simulink model "AC_Vfinal"  (R2019b)
settings: Solver=VariableStepAuto  StartTime=0.0  StopTime=sim_time  RelTol=1e-3
undefined symbols (not defined in the file): a1, A1, a2, A2, Ao, Cp_C, Cp_E, Cpa, Cpe, cpl, cpr, cpr1, cpr2, cpv, D, f1, f2, hfg, hr1, hr2, Kf, Mf, Mfl, Mfv, mr, N, n, Nc, nv, P, Qps, Qs, sp1, Ta, Tin, Uo, V, v, Vh1, Vh2, vs, Wg, Wm
libraries: simulink_extras x13
settings Model: Creator=aravi  LastModifiedBy=aravi
settings DataIOCC: SaveFormat=StructureWithTime  ReturnWorkspaceOutputs=off

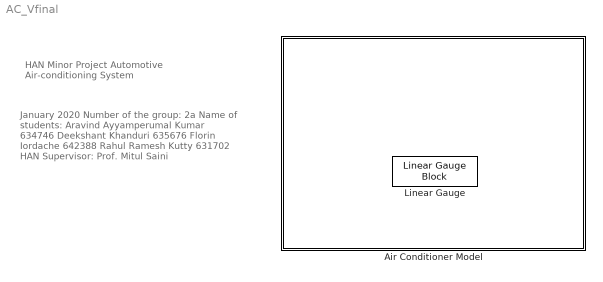
== system AC_Vfinal ==
  note: January 2020
      | Number of the group: 2a
      | Name of students:
      | Aravind Ayyamperumal Kumar 634746
      | Deekshant Khanduri 635676
      | Florin Iordache 642388
      | Rahul Ramesh Kutty 631702
      | HAN Supervisor: Prof. Mitul Saini
  note: HAN Minor Project
      | Automotive Air-conditioning System
  Air Conditioner Model : Subsystem
      mask Display: image('$imagefile'); % Use "Edit Image" on toolstrip to change.
  Linear Gauge : LinearGaugeBlock  ScaleMax=50  TickInterval=5

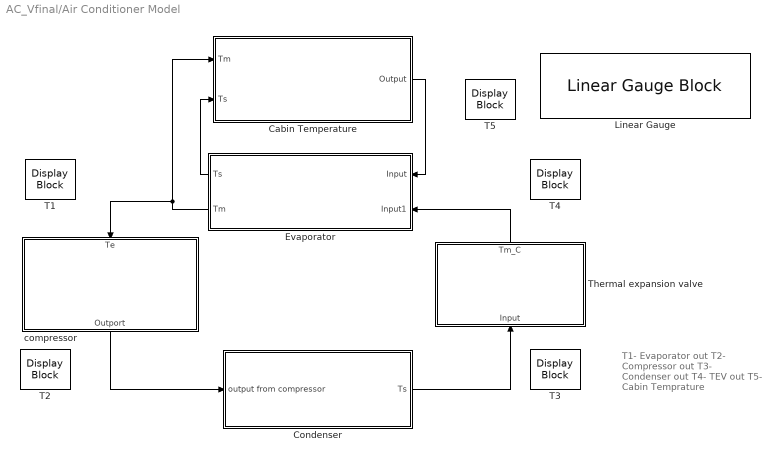
== system AC_Vfinal/Air Conditioner Model ==
  note: T1- Evaporator out
      | T2- Compressor out
      | T3- Condenser out
      | T4- TEV out
      | T5- Cabin Temprature
  Cabin Temperature : Subsystem
      mask Display: image('$imagefile'); % Use "Edit Image" on toolstrip to change.
  Condenser : Subsystem
      mask Display: image('$imagefile'); % Use "Edit Image" on toolstrip to change.
  Evaporator : Subsystem
      mask Display: image('$imagefile'); % Use "Edit Image" on toolstrip to change.
  Linear Gauge : LinearGaugeBlock  ScaleMax=50  TickInterval=5
  T{1..5} (5 alike) : DisplayBlock  LabelPosition=Hide  Format=short  Transparency=1
  Thermal expansion valve : Subsystem
      mask Display: image('$imagefile'); % Use "Edit Image" on toolstrip to change.
  compressor : Subsystem
      mask Display: image('$imagefile'); % Use "Edit Image" on toolstrip to change.
  wires:
  Evaporator/2(Tm) -> compressor/1(Te), Cabin Temperature/1(Tm)
  Condenser/1(Ts) -> Thermal expansion valve/1(Input)
  Cabin Temperature/1(Output) -> Evaporator/1(Input)
  compressor/1(Outport) -> Condenser/1(output from compressor)
  Thermal expansion valve/1(Tm_C) -> Evaporator/2(Input1)
  Evaporator/1(Ts) -> Cabin Temperature/2(Ts)

== system AC_Vfinal/Air Conditioner Model/Cabin Temperature ==
  Tm : Inport
  Ts : Inport  Port=2
  Temperature level : Subsystem
  Output : Outport
  wires:
  Tm/1 -> Temperature level/1(Tm)
  Temperature level/1(Output) -> Output/1
  Ts/1 -> Temperature level/2(Ts)

== system AC_Vfinal/Air Conditioner Model/Condenser ==
  output from compressor : Inport
  Mref : Subsystem
  Td block : Subsystem
  Tm block : Subsystem
  Ts block : Subsystem
  Tw block : Subsystem
  Ts : Outport
  wires:
  Ts block/2(Ts) -> Tw block/1(Ts)
  Tw block/1(Tw) -> Ts block/2(Tw), Td block/1(Tw)
  Td block/1(Td) -> Tw block/4(Td), Ts block/1(Td1)
  Ts block/1(Output to cabin Ts) -> Ts/1
  Tm block/1(Tm_C) -> Tw block/3(Tm), Td block/2(Tm)
  output from compressor/1 -> Tm block/1(Input)
  Mref/1(Out1) -> Tw block/2(Mref)

== system AC_Vfinal/Air Conditioner Model/Evaporator ==
  Input : Inport
  Input1 : Inport  Port=2
  Mref : Subsystem
  Td block : Subsystem
  Tm block : Subsystem
  Ts block : Subsystem
  Tw block : Subsystem
  Ts : Outport
  Tm : Outport  Port=2
  wires:
  Ts block/2(Ts) -> Tw block/1(Ts)
  Td block/1(Td) -> Tw block/4(Td), Ts block/1(Td1)
  Tw block/1(Tw) -> Ts block/2(Tw), Td block/1(Tw)
  Ts block/1(Output to cabin Ts) -> Ts/1
  Tm block/1(Tm_C) -> Tm/1, Tw block/3(Tm), Td block/2(Tm)
  Input/1 -> Tm block/1(Input)
  Input1/1 -> Tm block/2(Input1)
  Mref/1(Out1) -> Tw block/2(Mref)

== system AC_Vfinal/Air Conditioner Model/Thermal expansion valve ==
  note: Differential Equation
  note: Transfer Funtion
  note: Input
  note: process
  note: Output
  note: Input
  note: Process
  note: Output
  note: TinMfvcpv-ToutMflcpl = 0
  Input : Inport
  Gain1 : Gain  Gain=1/(Mfv*cpv)
  Gain4 : Gain  Gain=Mfl*cpl
  Input1 : InportShadow
  Scope : Scope
  Scope2 : Scope
  Transfer Fcn : TransferFcn  Numerator=[Mfl*cpl]  Denominator=[Mfv*cpv]
  Tm_C : Outport
  wires:
  Gain1/1 -> Scope2/1, Tm_C/1
  Input/1 -> Gain4/1
  Gain4/1 -> Gain1/1
  Transfer Fcn/1 -> Scope/1
  Input1/1 -> Transfer Fcn/1

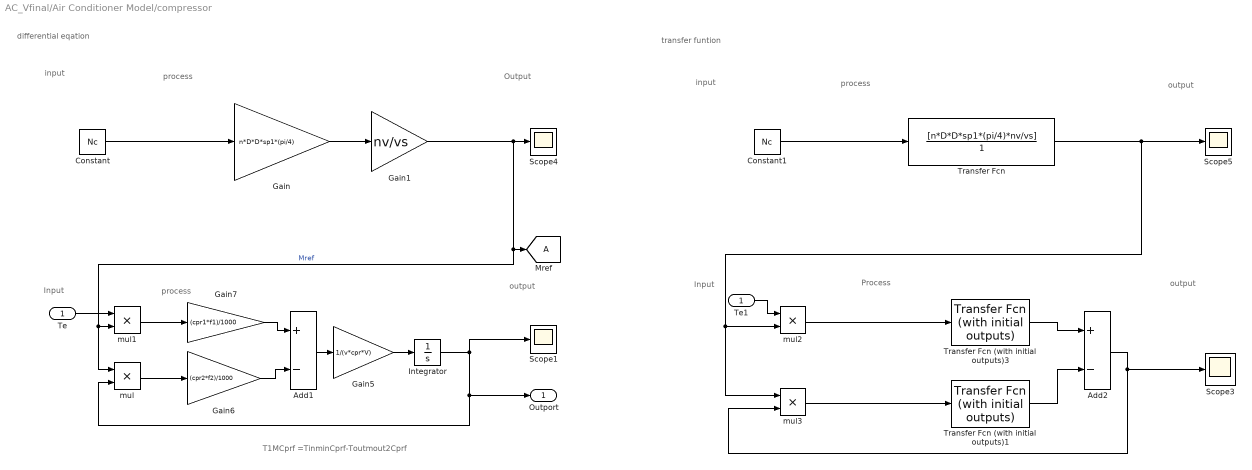
== system AC_Vfinal/Air Conditioner Model/compressor ==
  note: transfer funtion
  note: output
  note: process
  note: input
  note: output
  note: Process
  note: Input
  note: differential eqation
  note: input
  note: process
  note: Output
  note: process
  note: Input
  note: output
  note: T1MCprf =TinminCprf-Toutmout2Cprf
  Te : Inport
  Add1 : Sum  Inputs=+-
  Add2 : Sum  Inputs=+-
  Constant : Constant  Value=Nc  VectorParams1D=off  SampleTime=-1
  Constant1 : Constant  Value=Nc  VectorParams1D=off  SampleTime=-1
  Gain : Gain  Gain=n*D*D*sp1*(pi/4)
  Gain1 : Gain  Gain=nv/vs
  Gain5 : Gain  Gain=1/(v*cpr*V)
  Gain6 : Gain  Gain=(cpr2*f2)/1000
  Gain7 : Gain  Gain=(cpr1*f1)/1000
  Integrator : Integrator  InitialCondition=10
  Scope{1,3..5} (4 alike) : Scope
  Te1 : InportShadow
  Transfer Fcn : TransferFcn  Numerator=[n*D*D*sp1*(pi/4)*nv/vs]  Denominator=[1]
  Transfer Fcn (with initial outputs)1 : simulink_extras/Additional Linear/Transfer Fcn (with initial outputs)  N=[(cpr2*f2)/1000]  D=[v*cpr*V 0]  Y0=10  U0=27
  Transfer Fcn (with initial outputs)3 : simulink_extras/Additional Linear/Transfer Fcn (with initial outputs)  N=[(cpr1*f1)/1000]  D=[v*cpr*V 0]  Y0=20  U0=27
  mul{,1..3} (4 alike) : Product  Inputs=**
  Outport : Outport
  tag scope: A=global
  wires:
  Gain/1 -> Gain1/1
  Constant/1 -> Gain/1
  Integrator/1 -> Scope1/1, mul/2, Outport/1
  Add1/1 -> Gain5/1
  Gain6/1 -> Add1/2
  Gain7/1 -> Add1/1
  mul1/1 -> Gain7/1
  Gain5/1 -> Integrator/1
  Te/1 -> mul1/1
  Gain1/1 -> Scope4/1, [A], mul/1, mul1/2  "Mref"
  mul/1 -> Gain6/1
  Constant1/1 -> Transfer Fcn/1
  Transfer Fcn/1 -> Scope5/1, mul3/1, mul2/2
  mul2/1 -> Transfer Fcn (with initial outputs)3/1
  mul3/1 -> Transfer Fcn (with initial outputs)1/1
  Te1/1 -> mul2/1
  Transfer Fcn (with initial outputs)3/1 -> Add2/1
  Transfer Fcn (with initial outputs)1/1 -> Add2/2
  Add2/1 -> mul3/2, Scope3/1

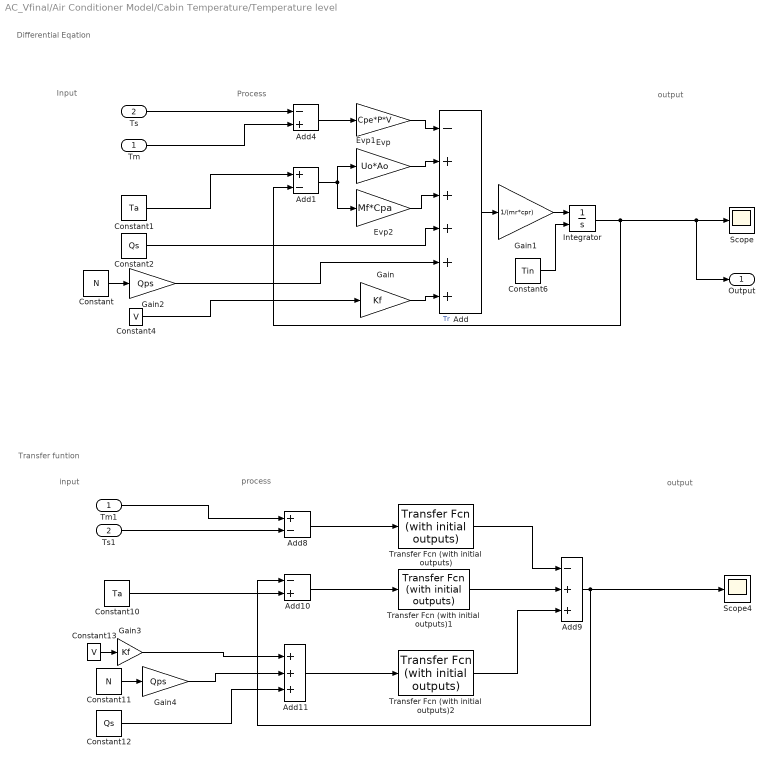
== system AC_Vfinal/Air Conditioner Model/Cabin Temperature/Temperature level ==
  note: Differential Eqation
  note: Input
  note: Process
  note: output
  note: Transfer funtion
  note: input
  note: process
  note: output
  Tm : Inport
  Ts : Inport  Port=2
  Add : Sum  Inputs=-+++++
  Add1 : Sum  Inputs=+-
  Add10 : Sum  Inputs=-+
  Add11 : Sum  Inputs=+++
  Add4 : Sum  Inputs=-+
  Add8 : Sum  Inputs=+-
  Add9 : Sum  Inputs=-++
  Constant : Constant  Value=N
  Constant1 : Constant  Value=Ta
  Constant10 : Constant  Value=Ta
  Constant11 : Constant  Value=N
  Constant12 : Constant  Value=Qs
  Constant13 : Constant  Value=V
  Constant2 : Constant  Value=Qs
  Constant4 : Constant  Value=V
  Constant6 : Constant  Value=Tin
  Evp : Gain  Gain=Cpe*P*V
  Evp1 : Gain  Gain=Uo*Ao
  Evp2 : Gain  Gain=Mf*Cpa
  Gain : Gain  Gain=Kf
  Gain1 : Gain  Gain=1/(mr*cpr)
  Gain2 : Gain  Gain=Qps
  Gain3 : Gain  Gain=Kf
  Gain4 : Gain  Gain=Qps
  Integrator : Integrator  InitialConditionSource=external
  Scope : Scope
  Scope4 : Scope
  Tm1 : InportShadow
  Transfer Fcn (with initial outputs) : simulink_extras/Additional Linear/Transfer Fcn (with initial outputs)  N=[Cpe*V*P]  D=[(mr*cpr) 0 ]  Y0=0  U0=27
  Transfer Fcn (with initial outputs)1 : simulink_extras/Additional Linear/Transfer Fcn (with initial outputs)  N=[Uo*Ao+Mf*Cpa]  D=[(mr*cpr) 0]  Y0=13.5  U0=28
  Transfer Fcn (with initial outputs)2 : simulink_extras/Additional Linear/Transfer Fcn (with initial outputs)  N=[1]  D=[(mr*cpr) 0 ]  Y0=13.5  U0=28
  Ts1 : InportShadow  Port=2
  Output : Outport
  wires:
  Gain1/1 -> Integrator/1
  Constant2/1 -> Add/4
  Constant4/1 -> Gain/1
  Constant/1 -> Gain2/1
  Constant6/1 -> Integrator/2
  Evp1/1 -> Add/2
  Evp2/1 -> Add/3
  Gain/1 -> Add/6
  Evp/1 -> Add/1
  Add/1 -> Gain1/1
  Integrator/1 -> Add1/2, Output/1, Scope/1  "Tr"
  Add1/1 -> Evp2/1, Evp1/1
  Add4/1 -> Evp/1
  Constant1/1 -> Add1/1
  Tm/1 -> Add4/2
  Ts/1 -> Add4/1
  Gain3/1 -> Add11/1
  Transfer Fcn (with initial outputs)1/1 -> Add9/2
  Transfer Fcn (with initial outputs)/1 -> Add9/1
  Constant12/1 -> Add11/3
  Constant13/1 -> Gain3/1
  Transfer Fcn (with initial outputs)2/1 -> Add9/3
  Constant11/1 -> Gain4/1
  Add8/1 -> Transfer Fcn (with initial outputs)/1
  Tm1/1 -> Add8/1
  Ts1/1 -> Add8/2
  Add10/1 -> Transfer Fcn (with initial outputs)1/1
  Add9/1 -> Scope4/1, Add10/1
  Add11/1 -> Transfer Fcn (with initial outputs)2/1
  Constant10/1 -> Add10/2
  Gain2/1 -> Add/5
  Gain4/1 -> Add11/2

== system AC_Vfinal/Air Conditioner Model/Condenser/Mref ==
  Multiply : Gain  Gain=1/10
  Out1 : Outport
  wires:
  [A] -> Multiply/1
  Multiply/1 -> Out1/1

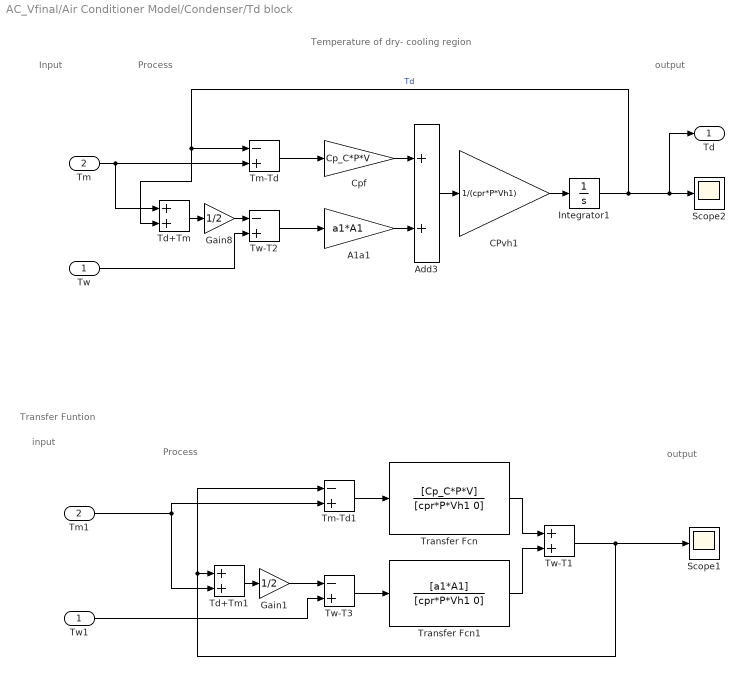
== system AC_Vfinal/Air Conditioner Model/Condenser/Td block ==
  note: Transfer Funtion
  note: output
  note: Process
  note: input
  note: Input
  note: Process
  note: output
  note: Temperature of dry- cooling region
  Tw : Inport
  Tm : Inport  Port=2
  A1a1 : Gain  Gain=a1*A1
  Add3 : Sum
  CPvh1 : Gain  Gain=1/(cpr*P*Vh1)
  Cpf : Gain  Gain=Cp_C*P*V
  Gain1 : Gain  Gain=1/2
  Gain8 : Gain  Gain=1/2
  Integrator1 : Integrator
  Scope1 : Scope
  Scope2 : Scope
  Td+Tm : Sum
  Td+Tm1 : Sum
  Tm-Td : Sum  Inputs=-+
  Tm-Td1 : Sum  Inputs=-+
  Tm1 : InportShadow  Port=2
  Transfer Fcn : TransferFcn  Numerator=[Cp_C*P*V]  Denominator=[cpr*P*Vh1 0]
  Transfer Fcn1 : TransferFcn  Numerator=[a1*A1]  Denominator=[cpr*P*Vh1 0]
  Tw-T1 : Sum
  Tw-T2 : Sum  Inputs=-+
  Tw-T3 : Sum  Inputs=-+
  Tw1 : InportShadow
  Td : Outport
  wires:
  Gain8/1 -> Tw-T2/1
  CPvh1/1 -> Integrator1/1
  Cpf/1 -> Add3/1
  Td+Tm/1 -> Gain8/1
  Tm-Td/1 -> Cpf/1
  Add3/1 -> CPvh1/1
  Integrator1/1 -> Td+Tm/2, Tm-Td/1, Td/1, Scope2/1  "Td"
  A1a1/1 -> Add3/2
  Tw-T2/1 -> A1a1/1
  Tw/1 -> Tw-T2/2
  Tm/1 -> Td+Tm/1, Tm-Td/2
  Transfer Fcn/1 -> Tw-T1/1
  Transfer Fcn1/1 -> Tw-T1/2
  Tw-T1/1 -> Tm-Td1/1, Td+Tm1/1, Scope1/1
  Tw-T3/1 -> Transfer Fcn1/1
  Tm-Td1/1 -> Transfer Fcn/1
  Gain1/1 -> Tw-T3/1
  Td+Tm1/1 -> Gain1/1
  Tw1/1 -> Tw-T3/2
  Tm1/1 -> Tm-Td1/2, Td+Tm1/2

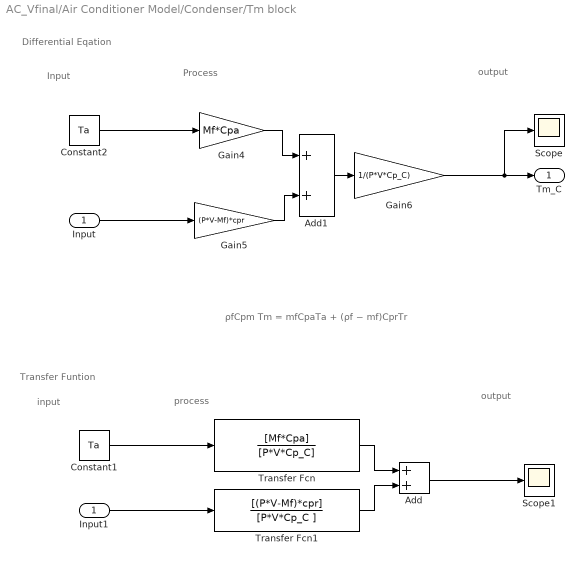
== system AC_Vfinal/Air Conditioner Model/Condenser/Tm block ==
  note: Differential Eqation
  note: Transfer Funtion
  note: output
  note: process
  note: input
  note: Process
  note: ρfCpm Tm = mfCpaTa + (ρf − mf)CprTr
  note: output
  note: Input
  Input : Inport
  Add : Sum
  Add1 : Sum
  Constant1 : Constant  Value=Ta
  Constant2 : Constant  Value=Ta
  Gain4 : Gain  Gain=Mf*Cpa
  Gain5 : Gain  Gain=(P*V-Mf)*cpr
  Gain6 : Gain  Gain=1/(P*V*Cp_C)
  Input1 : InportShadow
  Scope : Scope
  Scope1 : Scope
  Transfer Fcn : TransferFcn  Numerator=[Mf*Cpa]  Denominator=[P*V*Cp_C]
  Transfer Fcn1 : TransferFcn  Numerator=[(P*V-Mf)*cpr]  Denominator=[P*V*Cp_C ]
  Tm_C : Outport
  wires:
  Gain5/1 -> Add1/2
  Add1/1 -> Gain6/1
  Constant2/1 -> Gain4/1
  Gain6/1 -> Scope/1, Tm_C/1
  Gain4/1 -> Add1/1
  Add/1 -> Scope1/1
  Input/1 -> Gain5/1
  Constant1/1 -> Transfer Fcn/1
  Transfer Fcn/1 -> Add/1
  Transfer Fcn1/1 -> Add/2
  Input1/1 -> Transfer Fcn1/1

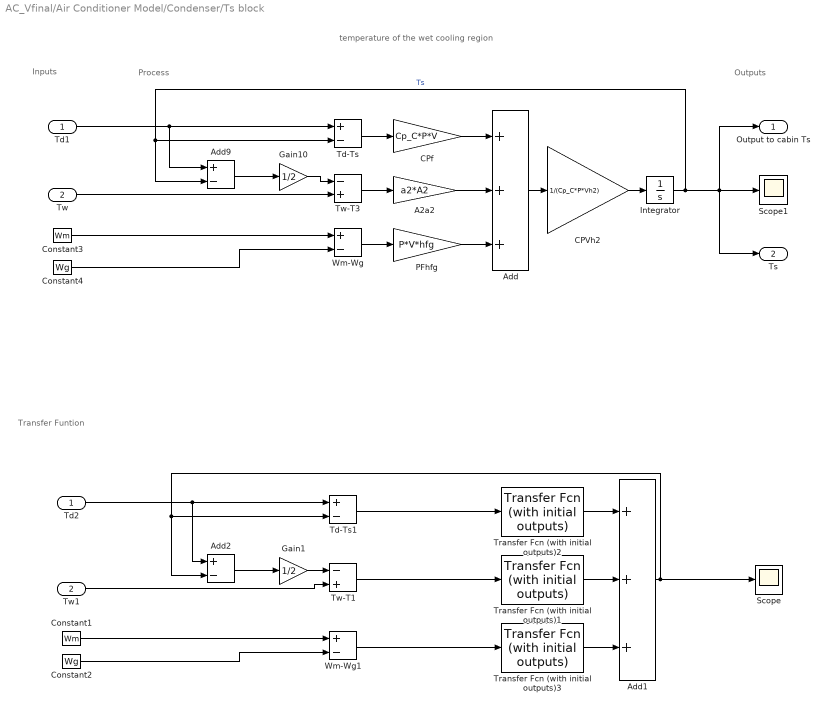
== system AC_Vfinal/Air Conditioner Model/Condenser/Ts block ==
  note: Transfer Funtion
  note: Inputs
  note: Process
  note: Outputs
  note: temperature of the wet cooling region
  Td1 : Inport
  Tw : Inport  Port=2
  A2a2 : Gain  Gain=a2*A2
  Add : Sum  Inputs=+++
  Add1 : Sum  Inputs=+++
  Add2 : Sum  Inputs=+-
  Add9 : Sum  Inputs=+-
  CPVh2 : Gain  Gain=1/(Cp_C*P*Vh2)
  CPf : Gain  Gain=Cp_C*P*V
  Constant1 : Constant  Value=Wm
  Constant2 : Constant  Value=Wg
  Constant3 : Constant  Value=Wm
  Constant4 : Constant  Value=Wg
  Gain1 : Gain  Gain=1/2
  Gain10 : Gain  Gain=1/2
  Integrator : Integrator  InitialCondition=27
  PFhfg : Gain  Gain=P*V*hfg
  Scope : Scope
  Scope1 : Scope
  Td-Ts : Sum  Inputs=+-
  Td-Ts1 : Sum  Inputs=+-
  Td2 : InportShadow
  Transfer Fcn (with initial outputs)1 : simulink_extras/Additional Linear/Transfer Fcn (with initial outputs)  N=[a2*A2]  D=[Cp_C*P*Vh2 0]  Y0=9  U0=27
  Transfer Fcn (with initial outputs)2 : simulink_extras/Additional Linear/Transfer Fcn (with initial outputs)  N=[Cp_C*P*V]  D=[Cp_C*P*Vh2 0]  Y0=9  U0=27
  Transfer Fcn (with initial outputs)3 : simulink_extras/Additional Linear/Transfer Fcn (with initial outputs)  N=[P*V*hfg]  D=[Cp_C*P*Vh2 0]  Y0=9  U0=27
  Tw-T1 : Sum  Inputs=-+
  Tw-T3 : Sum  Inputs=-+
  Tw1 : InportShadow  Port=2
  Wm-Wg : Sum  Inputs=+-
  Wm-Wg1 : Sum  Inputs=+-
  Output to cabin Ts : Outport
  Ts : Outport  Port=2
  wires:
  Constant3/1 -> Wm-Wg/1
  CPVh2/1 -> Integrator/1
  Integrator/1 -> Add9/2, Td-Ts/2, Output to cabin Ts/1, Scope1/1, Ts/1  "Ts"
  Add/1 -> CPVh2/1
  Constant4/1 -> Wm-Wg/2
  CPf/1 -> Add/1
  Wm-Wg/1 -> PFhfg/1
  Gain10/1 -> Tw-T3/1
  Td1/1 -> Add9/1, Td-Ts/1
  Tw-T3/1 -> A2a2/1
  Tw/1 -> Tw-T3/2
  Add9/1 -> Gain10/1
  Td-Ts/1 -> CPf/1
  A2a2/1 -> Add/2
  PFhfg/1 -> Add/3
  Transfer Fcn (with initial outputs)2/1 -> Add1/1
  Transfer Fcn (with initial outputs)1/1 -> Add1/2
  Transfer Fcn (with initial outputs)3/1 -> Add1/3
  Add1/1 -> Add2/2, Td-Ts1/2, Scope/1
  Wm-Wg1/1 -> Transfer Fcn (with initial outputs)3/1
  Tw-T1/1 -> Transfer Fcn (with initial outputs)1/1
  Td-Ts1/1 -> Transfer Fcn (with initial outputs)2/1
  Gain1/1 -> Tw-T1/1
  Add2/1 -> Gain1/1
  Tw1/1 -> Tw-T1/2
  Constant1/1 -> Wm-Wg1/1
  Constant2/1 -> Wm-Wg1/2
  Td2/1 -> Add2/1, Td-Ts1/1

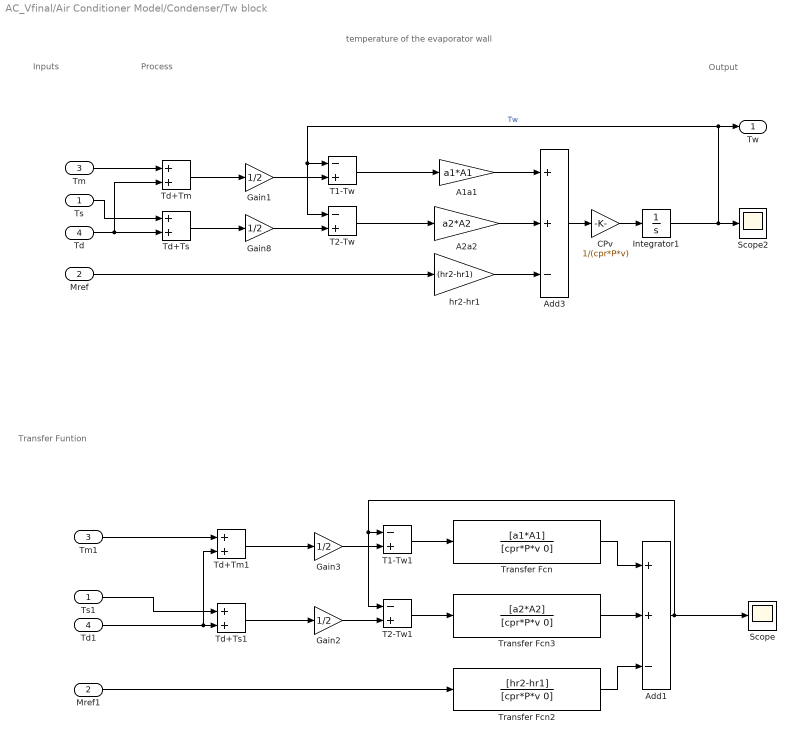
== system AC_Vfinal/Air Conditioner Model/Condenser/Tw block ==
  note: Transfer Funtion
  note: Inputs
  note: Process
  note: Output
  note: temperature of the evaporator wall
  Ts : Inport
  Mref : Inport  Port=2
  Tm : Inport  Port=3
  Td : Inport  Port=4
  A1a1 : Gain  Gain=a1*A1
  A2a2 : Gain  Gain=a2*A2
  Add1 : Sum  Inputs=++-
  Add3 : Sum  Inputs=++-
  CPv : Gain  Gain=1/(cpr*P*v)
  Gain{1..3,8} (4 alike) : Gain  Gain=1/2
  Integrator1 : Integrator  InitialCondition=28
  Mref1 : InportShadow  Port=2
  Scope : Scope
  Scope2 : Scope
  T1-Tw : Sum  Inputs=-+
  T1-Tw1 : Sum  Inputs=-+
  T2-Tw : Sum  Inputs=-+
  T2-Tw1 : Sum  Inputs=-+
  Td+Tm : Sum
  Td+Tm1 : Sum
  Td+Ts : Sum
  Td+Ts1 : Sum
  Td1 : InportShadow  Port=4
  Tm1 : InportShadow  Port=3
  Transfer Fcn : TransferFcn  Numerator=[a1*A1]  Denominator=[cpr*P*v 0]
  Transfer Fcn2 : TransferFcn  Numerator=[hr2-hr1]  Denominator=[cpr*P*v 0]
  Transfer Fcn3 : TransferFcn  Numerator=[a2*A2]  Denominator=[cpr*P*v 0]
  Ts1 : InportShadow
  hr2-hr1 : Gain  Gain=(hr2-hr1)
  Tw : Outport
  wires:
  T2-Tw/1 -> A2a2/1
  A2a2/1 -> Add3/2
  Integrator1/1 -> Scope2/1, T1-Tw/1, T2-Tw/1, Tw/1  "Tw"
  Add3/1 -> CPv/1
  T1-Tw/1 -> A1a1/1
  A1a1/1 -> Add3/1
  CPv/1 -> Integrator1/1
  Gain1/1 -> T1-Tw/2
  Td/1 -> Td+Tm/2, Td+Ts/2
  Gain8/1 -> T2-Tw/2
  Ts/1 -> Td+Ts/1
  Td+Tm/1 -> Gain1/1
  Td+Ts/1 -> Gain8/1
  hr2-hr1/1 -> Add3/3
  Tm/1 -> Td+Tm/1
  Transfer Fcn/1 -> Add1/1
  Transfer Fcn3/1 -> Add1/2
  Transfer Fcn2/1 -> Add1/3
  Add1/1 -> T2-Tw1/1, T1-Tw1/1, Scope/1
  T2-Tw1/1 -> Transfer Fcn3/1
  T1-Tw1/1 -> Transfer Fcn/1
  Mref1/1 -> Transfer Fcn2/1
  Gain2/1 -> T2-Tw1/2
  Td+Ts1/1 -> Gain2/1
  Td+Tm1/1 -> Gain3/1
  Gain3/1 -> T1-Tw1/2
  Tm1/1 -> Td+Tm1/1
  Td1/1 -> Td+Tm1/2, Td+Ts1/2
  Ts1/1 -> Td+Ts1/1
  Mref/1 -> hr2-hr1/1

== system AC_Vfinal/Air Conditioner Model/Evaporator/Mref ==
  Gain : Gain  Gain=1/100
  Out1 : Outport
  wires:
  [A] -> Gain/1
  Gain/1 -> Out1/1

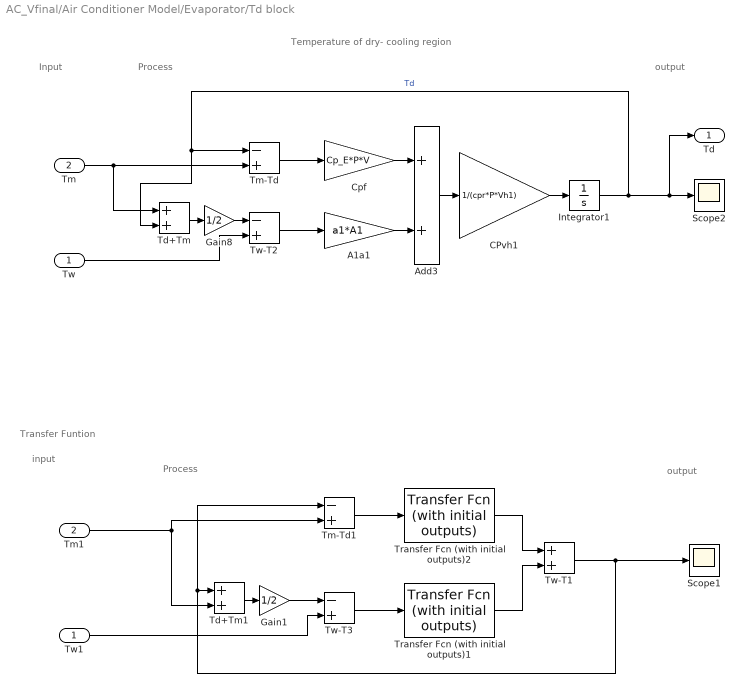
== system AC_Vfinal/Air Conditioner Model/Evaporator/Td block ==
  note: Input
  note: Process
  note: output
  note: Temperature of dry- cooling region
  note: output
  note: Transfer Funtion
  note: input
  note: Process
  Tw : Inport
  Tm : Inport  Port=2
  A1a1 : Gain  Gain=a1*A1
  Add3 : Sum
  CPvh1 : Gain  Gain=1/(cpr*P*Vh1)
  Cpf : Gain  Gain=Cp_E*P*V
  Gain1 : Gain  Gain=1/2
  Gain8 : Gain  Gain=1/2
  Integrator1 : Integrator  InitialCondition=27
  Scope1 : Scope
  Scope2 : Scope
  Td+Tm : Sum
  Td+Tm1 : Sum
  Tm-Td : Sum  Inputs=-+
  Tm-Td1 : Sum  Inputs=-+
  Tm1 : InportShadow  Port=2
  Transfer Fcn (with initial outputs)1 : simulink_extras/Additional Linear/Transfer Fcn (with initial outputs)  N=[a1*A1]  D=[cpr*P*Vh1 0]  Y0=9  U0=27
  Transfer Fcn (with initial outputs)2 : simulink_extras/Additional Linear/Transfer Fcn (with initial outputs)  N=[Cp_E*P*V]  D=[cpr*P*Vh1 0]  Y0=9  U0=27
  Tw-T1 : Sum
  Tw-T2 : Sum  Inputs=-+
  Tw-T3 : Sum  Inputs=-+
  Tw1 : InportShadow
  Td : Outport
  wires:
  Gain8/1 -> Tw-T2/1
  CPvh1/1 -> Integrator1/1
  Cpf/1 -> Add3/1
  Td+Tm/1 -> Gain8/1
  Tm-Td/1 -> Cpf/1
  Add3/1 -> CPvh1/1
  Integrator1/1 -> Td+Tm/2, Tm-Td/1, Td/1, Scope2/1  "Td"
  A1a1/1 -> Add3/2
  Tw-T2/1 -> A1a1/1
  Tw/1 -> Tw-T2/2
  Tm/1 -> Td+Tm/1, Tm-Td/2
  Tm-Td1/1 -> Transfer Fcn (with initial outputs)2/1
  Transfer Fcn (with initial outputs)2/1 -> Tw-T1/1
  Gain1/1 -> Tw-T3/1
  Tw1/1 -> Tw-T3/2
  Tw-T3/1 -> Transfer Fcn (with initial outputs)1/1
  Tm1/1 -> Tm-Td1/2, Td+Tm1/2
  Tw-T1/1 -> Tm-Td1/1, Td+Tm1/1, Scope1/1
  Transfer Fcn (with initial outputs)1/1 -> Tw-T1/2
  Td+Tm1/1 -> Gain1/1

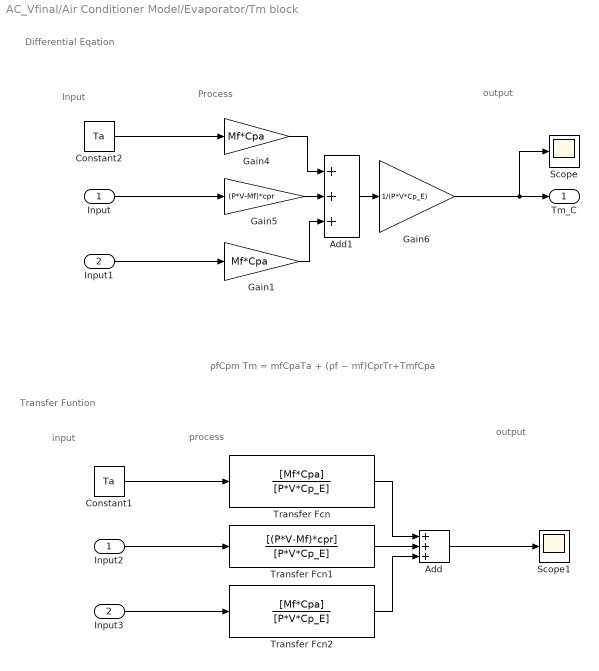
== system AC_Vfinal/Air Conditioner Model/Evaporator/Tm block ==
  note: Differential Eqation
  note: Process
  note: ρfCpm Tm = mfCpaTa + (ρf − mf)CprTr+TmfCpa
  note: output
  note: Input
  note: input
  note: process
  note: output
  note: Transfer Funtion
  Input : Inport
  Input1 : Inport  Port=2
  Add : Sum  Inputs=+++
  Add1 : Sum  Inputs=+++
  Constant1 : Constant  Value=Ta
  Constant2 : Constant  Value=Ta
  Gain1 : Gain  Gain=Mf*Cpa
  Gain4 : Gain  Gain=Mf*Cpa
  Gain5 : Gain  Gain=(P*V-Mf)*cpr
  Gain6 : Gain  Gain=1/(P*V*Cp_E)
  Input2 : InportShadow
  Input3 : InportShadow  Port=2
  Scope : Scope
  Scope1 : Scope
  Transfer Fcn : TransferFcn  Numerator=[Mf*Cpa]  Denominator=[P*V*Cp_E]
  Transfer Fcn1 : TransferFcn  Numerator=[(P*V-Mf)*cpr]  Denominator=[P*V*Cp_E]
  Transfer Fcn2 : TransferFcn  Numerator=[Mf*Cpa]  Denominator=[P*V*Cp_E]
  Tm_C : Outport
  wires:
  Gain5/1 -> Add1/2
  Add1/1 -> Gain6/1
  Input/1 -> Gain5/1
  Constant2/1 -> Gain4/1
  Gain6/1 -> Scope/1, Tm_C/1
  Gain4/1 -> Add1/1
  Input1/1 -> Gain1/1
  Gain1/1 -> Add1/3
  Constant1/1 -> Transfer Fcn/1
  Transfer Fcn1/1 -> Add/2
  Transfer Fcn/1 -> Add/1
  Add/1 -> Scope1/1
  Input2/1 -> Transfer Fcn1/1
  Transfer Fcn2/1 -> Add/3
  Input3/1 -> Transfer Fcn2/1

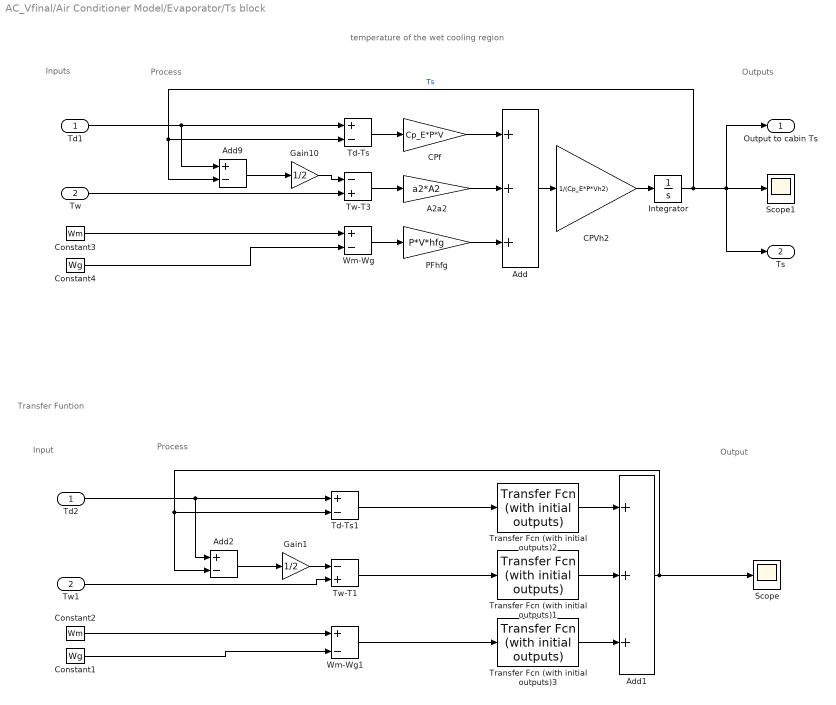
== system AC_Vfinal/Air Conditioner Model/Evaporator/Ts block ==
  note: Inputs
  note: Process
  note: Outputs
  note: temperature of the wet cooling region
  note: Input
  note: Transfer Funtion
  note: Process
  note: Output
  Td1 : Inport
  Tw : Inport  Port=2
  A2a2 : Gain  Gain=a2*A2
  Add : Sum  Inputs=+++
  Add1 : Sum  Inputs=+++
  Add2 : Sum  Inputs=+-
  Add9 : Sum  Inputs=+-
  CPVh2 : Gain  Gain=1/(Cp_E*P*Vh2)
  CPf : Gain  Gain=Cp_E*P*V
  Constant1 : Constant  Value=Wg
  Constant2 : Constant  Value=Wm
  Constant3 : Constant  Value=Wm
  Constant4 : Constant  Value=Wg
  Gain1 : Gain  Gain=1/2
  Gain10 : Gain  Gain=1/2
  Integrator : Integrator  InitialCondition=27
  PFhfg : Gain  Gain=P*V*hfg
  Scope : Scope
  Scope1 : Scope
  Td-Ts : Sum  Inputs=+-
  Td-Ts1 : Sum  Inputs=+-
  Td2 : InportShadow
  Transfer Fcn (with initial outputs)1 : simulink_extras/Additional Linear/Transfer Fcn (with initial outputs)  N=[a2*A2]  D=[Cp_E*P*Vh2 0]  Y0=9  U0=27
  Transfer Fcn (with initial outputs)2 : simulink_extras/Additional Linear/Transfer Fcn (with initial outputs)  N=[Cp_E*P*V]  D=[Cp_E*P*Vh2 0]  Y0=9  U0=27
  Transfer Fcn (with initial outputs)3 : simulink_extras/Additional Linear/Transfer Fcn (with initial outputs)  N=[P*V*hfg]  D=[Cp_E*P*Vh2 0]  Y0=9  U0=27
  Tw-T1 : Sum  Inputs=-+
  Tw-T3 : Sum  Inputs=-+
  Tw1 : InportShadow  Port=2
  Wm-Wg : Sum  Inputs=+-
  Wm-Wg1 : Sum  Inputs=+-
  Output to cabin Ts : Outport
  Ts : Outport  Port=2
  wires:
  Constant3/1 -> Wm-Wg/1
  CPVh2/1 -> Integrator/1
  Integrator/1 -> Add9/2, Td-Ts/2, Output to cabin Ts/1, Scope1/1, Ts/1  "Ts"
  Add/1 -> CPVh2/1
  Constant4/1 -> Wm-Wg/2
  CPf/1 -> Add/1
  Wm-Wg/1 -> PFhfg/1
  Gain10/1 -> Tw-T3/1
  Td1/1 -> Add9/1, Td-Ts/1
  Tw-T3/1 -> A2a2/1
  Tw/1 -> Tw-T3/2
  Add9/1 -> Gain10/1
  Td-Ts/1 -> CPf/1
  A2a2/1 -> Add/2
  PFhfg/1 -> Add/3
  Gain1/1 -> Tw-T1/1
  Transfer Fcn (with initial outputs)3/1 -> Add1/3
  Add1/1 -> Add2/2, Td-Ts1/2, Scope/1
  Transfer Fcn (with initial outputs)2/1 -> Add1/1
  Constant2/1 -> Wm-Wg1/1
  Add2/1 -> Gain1/1
  Td2/1 -> Add2/1, Td-Ts1/1
  Tw-T1/1 -> Transfer Fcn (with initial outputs)1/1
  Constant1/1 -> Wm-Wg1/2
  Transfer Fcn (with initial outputs)1/1 -> Add1/2
  Wm-Wg1/1 -> Transfer Fcn (with initial outputs)3/1
  Td-Ts1/1 -> Transfer Fcn (with initial outputs)2/1
  Tw1/1 -> Tw-T1/2

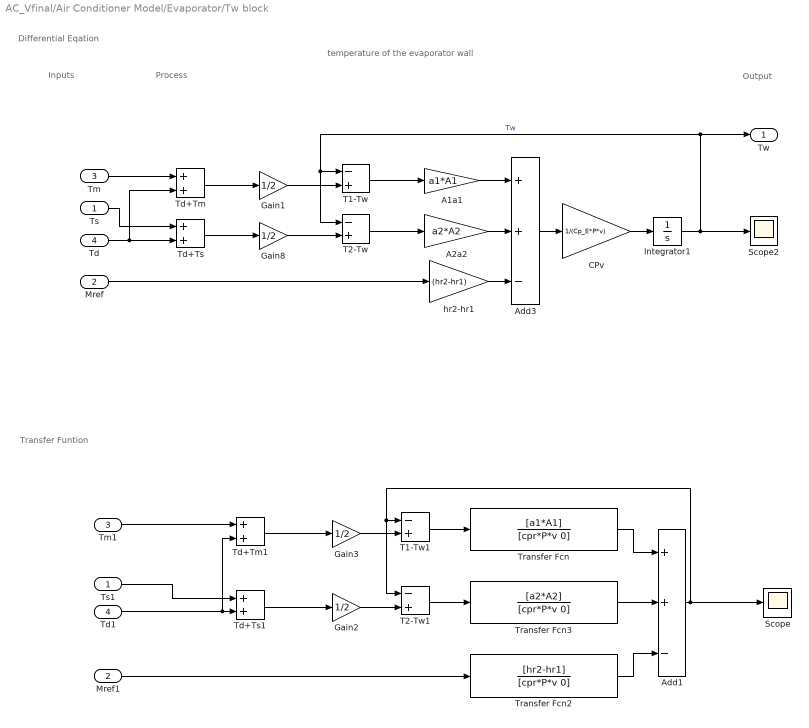
== system AC_Vfinal/Air Conditioner Model/Evaporator/Tw block ==
  note: Differential Eqation
  note: Inputs
  note: Process
  note: Output
  note: temperature of the evaporator wall
  note: Transfer Funtion
  Ts : Inport
  Mref : Inport  Port=2
  Tm : Inport  Port=3
  Td : Inport  Port=4
  A1a1 : Gain  Gain=a1*A1
  A2a2 : Gain  Gain=a2*A2
  Add1 : Sum  Inputs=++-
  Add3 : Sum  Inputs=++-
  CPv : Gain  Gain=1/(Cp_E*P*v)
  Gain{1..3,8} (4 alike) : Gain  Gain=1/2
  Integrator1 : Integrator  InitialCondition=28
  Mref1 : InportShadow  Port=2
  Scope : Scope
  Scope2 : Scope
  T1-Tw : Sum  Inputs=-+
  T1-Tw1 : Sum  Inputs=-+
  T2-Tw : Sum  Inputs=-+
  T2-Tw1 : Sum  Inputs=-+
  Td+Tm : Sum
  Td+Tm1 : Sum
  Td+Ts : Sum
  Td+Ts1 : Sum
  Td1 : InportShadow  Port=4
  Tm1 : InportShadow  Port=3
  Transfer Fcn : TransferFcn  Numerator=[a1*A1]  Denominator=[cpr*P*v 0]
  Transfer Fcn2 : TransferFcn  Numerator=[hr2-hr1]  Denominator=[cpr*P*v 0]
  Transfer Fcn3 : TransferFcn  Numerator=[a2*A2]  Denominator=[cpr*P*v 0]
  Ts1 : InportShadow
  hr2-hr1 : Gain  Gain=(hr2-hr1)
  Tw : Outport
  wires:
  T2-Tw/1 -> A2a2/1
  A2a2/1 -> Add3/2
  Integrator1/1 -> Scope2/1, Tw/1, T1-Tw/1, T2-Tw/1  "Tw"
  Add3/1 -> CPv/1
  T1-Tw/1 -> A1a1/1
  A1a1/1 -> Add3/1
  CPv/1 -> Integrator1/1
  Gain1/1 -> T1-Tw/2
  Td/1 -> Td+Tm/2, Td+Ts/2
  Gain8/1 -> T2-Tw/2
  Ts/1 -> Td+Ts/1
  Td+Tm/1 -> Gain1/1
  Td+Ts/1 -> Gain8/1
  hr2-hr1/1 -> Add3/3
  Tm/1 -> Td+Tm/1
  Ts1/1 -> Td+Ts1/1
  T2-Tw1/1 -> Transfer Fcn3/1
  Mref1/1 -> Transfer Fcn2/1
  Gain2/1 -> T2-Tw1/2
  T1-Tw1/1 -> Transfer Fcn/1
  Gain3/1 -> T1-Tw1/2
  Td+Ts1/1 -> Gain2/1
  Tm1/1 -> Td+Tm1/1
  Transfer Fcn/1 -> Add1/1
  Td+Tm1/1 -> Gain3/1
  Transfer Fcn3/1 -> Add1/2
  Transfer Fcn2/1 -> Add1/3
  Add1/1 -> T2-Tw1/1, T1-Tw1/1, Scope/1
  Td1/1 -> Td+Tm1/2, Td+Ts1/2
  Mref/1 -> hr2-hr1/1
